simulink model "power_neutral"  (Simulink 6.0)
settings: Solver=VariableStepDiscrete  SolverMode=SingleTasking  StartTime=0.0  StopTime=10.0  MaxStep=1e-03  RelTol=1e-3  AbsTol=1e-6
libraries: powerlib x13
settings Model: Creator=patrice  LastModifiedBy=batserve  ExtModeTrigMode=oneshot  ExtModeArmWhenConnect=off  ExtModeAutoUpdateStatusClock=off
settings DataIOCC: LimitDataPoints=off  SignalLoggingName=sigsOut
settings OptimizationCC: BooleanDataType=off
settings DebuggingCC: SolverPrmCheckMsg=none
settings HardwareCC: TargetUnknown=on
settings RTWCC: TemplateMakefile=grt_unix.tmf

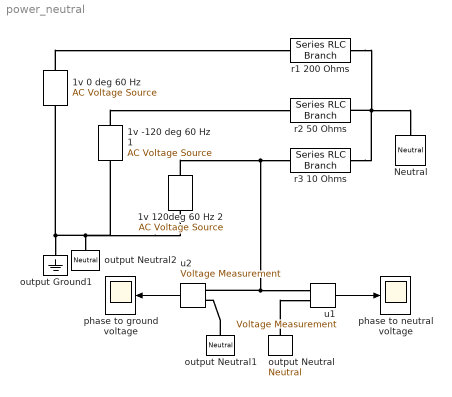
== system power_neutral ==
  1v -120 deg 60 Hz 1 : powerlib/Electrical Sources/AC Voltage Source  Description=source block  Orientation=up  Amplitude=1  Phase=-120  Frequency=60  SampleTime=0  Measurements=None
      settings: AttributesFormatString=\n
  "1v 0 deg 60 Hz " : powerlib/Electrical Sources/AC Voltage Source  Description=source block  Orientation=up  Amplitude=1  Phase=0  Frequency=60  SampleTime=0  Measurements=None
      settings: AttributesFormatString=\n
  1v 120deg 60 Hz 2 : powerlib/Electrical Sources/AC Voltage Source  Description=source block  Orientation=up  Amplitude=1  Phase=120  Frequency=60  SampleTime=0  Measurements=None
      settings: AttributesFormatString=\n
  Neutral : powerlib/Elements/Neutral  Orientation=down  PhysicalDomain=powersysdomain  SubClassName=unknown  PortType=p1  LConnTagsString=a  NodeNumber=50
  output Ground1 : powerlib/Elements/Ground  Orientation=down  PhysicalDomain=powersysdomain  SubClassName=unknown  PortType=p1  LConnTagsString=a
  output Neutral : powerlib/Elements/Neutral  Orientation=down  PhysicalDomain=powersysdomain  SubClassName=unknown  PortType=p1  LConnTagsString=a  NodeNumber=50
  output Neutral1 : powerlib/Elements/Neutral  Orientation=down  PhysicalDomain=powersysdomain  SubClassName=unknown  PortType=p1  LConnTagsString=a  NodeNumber=0
  output Neutral2 : powerlib/Elements/Neutral  Orientation=down  PhysicalDomain=powersysdomain  SubClassName=unknown  PortType=p1  LConnTagsString=a  NodeNumber=0
  phase to ground voltage : Scope
      settings: TickLabels=on  TimeRange=0.1  YMin=-1.2  YMax=1.2  DataFormat=Array
  phase to neutral voltage : Scope
      settings: TickLabels=on  TimeRange=0.1  YMin=-1.2  YMax=1.2  DataFormat=Array
  r1 200 Ohms : powerlib/Elements/Series RLC Branch  PhysicalDomain=powersysdomain  SubClassName=unknown  PortType=p1  LConnTagsString=__new0  RConnTagsString=__new0  Resistance=200  Inductance=0  Capacitance=inf  Measurements=None
  r2 50 Ohms : powerlib/Elements/Series RLC Branch  PhysicalDomain=powersysdomain  SubClassName=unknown  PortType=p1  LConnTagsString=__new0  RConnTagsString=__new0  Resistance=50  Inductance=0  Capacitance=inf  Measurements=None
  r3 10 Ohms : powerlib/Elements/Series RLC Branch  PhysicalDomain=powersysdomain  SubClassName=unknown  PortType=p1  LConnTagsString=__new0  RConnTagsString=__new0  Resistance=10  Inductance=0  Capacitance=inf  Measurements=None
  u1 : powerlib/Measurements/Voltage Measurement  Tag=PoWeRsYsTeMmEaSuReMeNt  PhasorSimulation=off  OutputType=Magnitude  PSBequivalent=0
  u2 : powerlib/Measurements/Voltage Measurement  Tag=PoWeRsYsTeMmEaSuReMeNt  Orientation=left  PhasorSimulation=off  OutputType=Magnitude  PSBequivalent=0
  wires:
  u1/1 -> phase to neutral voltage/1
  u2/1 -> phase to ground voltage/1
  connections:
  1v -120 deg 60 Hz 1/LConn1 -- 1v 120deg 60 Hz 2/LConn1 -- "1v 0 deg 60 Hz "/LConn1 -- output Ground1/LConn1 -- output Neutral2/LConn1
  "1v 0 deg 60 Hz "/RConn1 -- r1 200 Ohms/LConn1
  r1 200 Ohms/RConn1 -- r2 50 Ohms/RConn1 -- r3 10 Ohms/RConn1 -- Neutral/LConn1
  1v -120 deg 60 Hz 1/RConn1 -- r2 50 Ohms/LConn1
  output Neutral/LConn1 -- u1/LConn2
  output Neutral1/LConn1 -- u2/LConn2
  1v 120deg 60 Hz 2/RConn1 -- r3 10 Ohms/LConn1 -- u2/LConn1 -- u1/LConn1
